simulink library "GearLibrary"  (R2017b)
settings: Solver=VariableStepAuto  StartTime=0.0  StopTime=10.0  RelTol=1e-3
undefined symbols (not defined in the file): c_LTset, DiscIntNeverNeededParam, g, Gear, magnitude, Strut, Tss, x1_LTset
libraries: GearLibrary x11, BaseLibrary x6, simulink x4, MathLibrary x2, vrlib x1
(part 1 of 2)
settings Model: Creator=Holzapfel  LastModifiedBy=zht
settings CodeAppCC: StateflowObjectComments=on

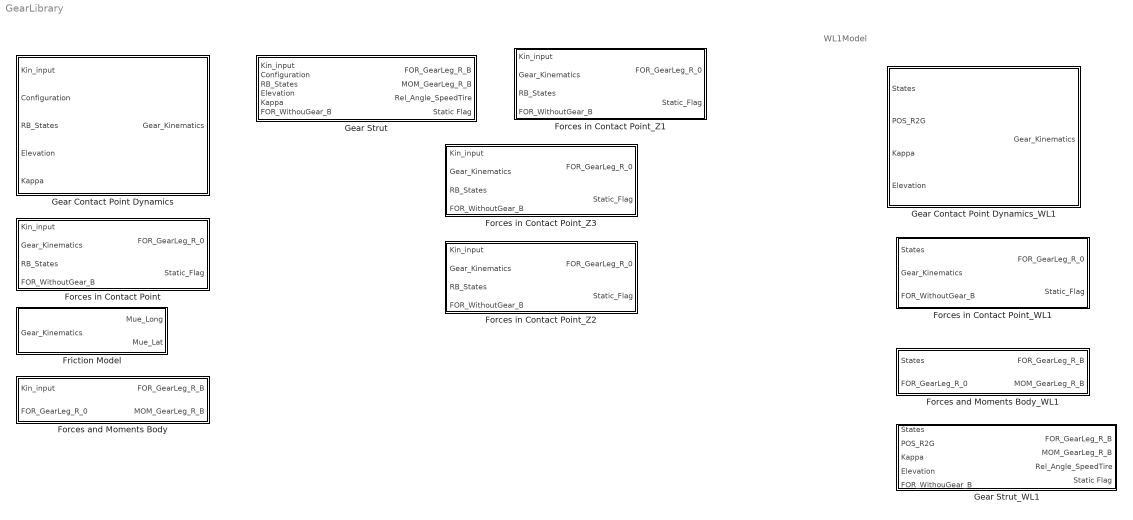
== system GearLibrary ==
  note: WL1Model
  Forces and Moments Body : Subsystem  mask{POS_R_GearStrut_B=Strut.POS_R_GearStrut_B}
      mask prompts: POS_R_GearStrut_B "POS R => Contact Point, Body Frame"
  Forces and Moments Body_WL1 : Subsystem  mask{POS_R_GearStrut_B=Strut.POS_R_GearStrut_B}
      mask prompts: POS_R_GearStrut_B "POS R => Contact Point, Body Frame"
  Forces in Contact Point : Subsystem  mask{h_StrutUndeflected=Strut.h_StrutUndeflected, c=Strut.c, d=Strut.d, ct=Strut.ct, dt=Strut.dt, FOR_MaxDamp=Strut.FOR_MaxDamp, FOR_MaxSpring=Strut.FOR_MaxSpring, Mue_Roll=Strut.Mue_Roll, Mue_Lat_per_Slip=Strut.Mue_Lat_per_Slip, Mue_Lat_Max=Strut.Mue_Lat_Max, Compress_LengthMax=Strut.Compress_LengthMax, Mue_Static=Strut.Mue_Static}
      mask prompts: h_StrutUndeflected "Length of undeflected landing gear strut [m]"; c "Strut Spring Constant [N/m]"; d "Strut Damping Constant [N/(m/s)]"; ct "Consider tire and ground is also a spring system, so it's Ground Spring Constant [N/m]"; dt "Consider tire and ground is also a spring system, so it's Ground Damping Constant [N/m]"; FOR_MaxDamp "Maximum Strut Damper Force [N]"; FOR_MaxSpring "Maximum Strut Spring Force [Nm]"; Mue_Roll "Rolling Friction Coefficient [-]"; Mue_Lat_per_Slip "Lateral Friction Coefficient per Slip Angle [1/rad]"; Mue_Lat_Max "Maximum Lateral Friction Coefficient [-]"; Compress_LengthMax "Maximum Compression length [m]"; Mue_Static "Static  Friction Coefficient"
  Forces in Contact Point_WL1 : Subsystem  mask{h_StrutUndeflected=Strut.h_StrutUndeflected, c=Strut.c, d=Strut.d, ct=Strut.ct, dt=Strut.dt, FOR_MaxDamp=Strut.FOR_MaxDamp, FOR_MaxSpring=Strut.FOR_MaxSpring, Mue_Roll=Strut.Mue_Roll, Mue_Lat_per_Slip=Strut.Mue_Lat_per_Slip, Mue_Lat_Max=Strut.Mue_Lat_Max, Compress_LengthMax=Strut.Compress_LengthMax, Mue_Static=Strut.Mue_Static, Compress_LengthMax_Tire=Strut.Compress_LengthMax_Tire}
      mask prompts: h_StrutUndeflected "Length of undeflected landing gear strut [m]"; c "Strut Spring Constant [N/m]"; d "Strut Damping Constant [N/(m/s)]"; ct "Consider tire and ground is also a spring system, so it's Ground Spring Constant [N/m]"; dt "Consider tire and ground is also a spring system, so it's Ground Damping Constant [N/m]"; FOR_MaxDamp "Maximum Strut Damper Force [N]"; FOR_MaxSpring "Maximum Strut Spring Force [Nm]"; Mue_Roll "Rolling Friction Coefficient [-]"; Mue_Lat_per_Slip "Lateral Friction Coefficient per Slip Angle [1/rad]"; Mue_Lat_Max "Maximum Lateral Friction Coefficient [-]"; Compress_LengthMax "Maximum Compression length [m]"; Mue_Static "Static  Friction Coefficient"; Compress_LengthMax_Tire "Maximum Compression length [m]"
  Forces in Contact Point_Z1 : Subsystem  mask{h_StrutUndeflected=Strut.h_StrutUndeflected, c=Strut.c, d=Strut.d, ct=Strut.ct, dt=Strut.dt, FOR_MaxDamp=Strut.FOR_MaxDamp, FOR_MaxSpring=Strut.FOR_MaxSpring, Mue_Roll=Strut.Mue_Roll, Mue_Lat_per_Slip=Strut.Mue_Lat_per_Slip, Mue_Lat_Max=Strut.Mue_Lat_Max, Compress_LengthMax=Strut.Compress_LengthMax, Mue_Static=Strut.Mue_Static, Compress_LengthMax_Tire=Strut.Compress_LengthMax_Tire}
      mask prompts: h_StrutUndeflected "Length of undeflected landing gear strut [m]"; c "Strut Spring Constant [N/m]"; d "Strut Damping Constant [N/(m/s)]"; ct "Consider tire and ground is also a spring system, so it's Ground Spring Constant [N/m]"; dt "Consider tire and ground is also a spring system, so it's Ground Damping Constant [N/m]"; FOR_MaxDamp "Maximum Strut Damper Force [N]"; FOR_MaxSpring "Maximum Strut Spring Force [Nm]"; Mue_Roll "Rolling Friction Coefficient [-]"; Mue_Lat_per_Slip "Lateral Friction Coefficient per Slip Angle [1/rad]"; Mue_Lat_Max "Maximum Lateral Friction Coefficient [-]"; Compress_LengthMax "Maximum Compression length [m]"; Mue_Static "Static  Friction Coefficient"; Compress_LengthMax_Tire "Maximum Compression length [m]"
  Forces in Contact Point_Z2 : Subsystem  mask{h_StrutUndeflected=Strut.h_StrutUndeflected, c=Strut.c, d=Strut.d, ct=Strut.ct, dt=Strut.dt, FOR_MaxDamp=Strut.FOR_MaxDamp, FOR_MaxSpring=Strut.FOR_MaxSpring, Mue_Roll=Strut.Mue_Roll, Mue_Lat_per_Slip=Strut.Mue_Lat_per_Slip, Mue_Lat_Max=Strut.Mue_Lat_Max, Compress_LengthMax=Strut.Compress_LengthMax, Mue_Static=Strut.Mue_Static, Compress_LengthMax_Tire=Strut.Compress_LengthMax_Tire}
      mask prompts: h_StrutUndeflected "Length of undeflected landing gear strut [m]"; c "Strut Spring Constant [N/m]"; d "Strut Damping Constant [N/(m/s)]"; ct "Consider tire and ground is also a spring system, so it's Ground Spring Constant [N/m]"; dt "Consider tire and ground is also a spring system, so it's Ground Damping Constant [N/m]"; FOR_MaxDamp "Maximum Strut Damper Force [N]"; FOR_MaxSpring "Maximum Strut Spring Force [Nm]"; Mue_Roll "Rolling Friction Coefficient [-]"; Mue_Lat_per_Slip "Lateral Friction Coefficient per Slip Angle [1/rad]"; Mue_Lat_Max "Maximum Lateral Friction Coefficient [-]"; Compress_LengthMax "Maximum Compression length [m]"; Mue_Static "Static  Friction Coefficient"; Compress_LengthMax_Tire "Maximum Compression length [m]"
  Forces in Contact Point_Z3 : Subsystem  mask{h_StrutUndeflected=Strut.h_StrutUndeflected, c=Strut.c, d=Strut.d, ct=Strut.ct, dt=Strut.dt, FOR_MaxDamp=Strut.FOR_MaxDamp, FOR_MaxSpring=Strut.FOR_MaxSpring, Mue_Roll=Strut.Mue_Roll, Mue_Lat_per_Slip=Strut.Mue_Lat_per_Slip, Mue_Lat_Max=Strut.Mue_Lat_Max, Compress_LengthMax=Strut.Compress_LengthMax, Mue_Static=Strut.Mue_Static}
      mask prompts: h_StrutUndeflected "Length of undeflected landing gear strut [m]"; c "Strut Spring Constant [N/m]"; d "Strut Damping Constant [N/(m/s)]"; ct "Consider tire and ground is also a spring system, so it's Ground Spring Constant [N/m]"; dt "Consider tire and ground is also a spring system, so it's Ground Damping Constant [N/m]"; FOR_MaxDamp "Maximum Strut Damper Force [N]"; FOR_MaxSpring "Maximum Strut Spring Force [Nm]"; Mue_Roll "Rolling Friction Coefficient [-]"; Mue_Lat_per_Slip "Lateral Friction Coefficient per Slip Angle [1/rad]"; Mue_Lat_Max "Maximum Lateral Friction Coefficient [-]"; Compress_LengthMax "Maximum Compression length [m]"; Mue_Static "Static  Friction Coefficient"
  Friction Model : Subsystem  mask{Mue_Roll=Strut.Mue_Roll, Mue_Lat_per_Slip=Strut.Mue_Lat_per_Slip, Mue_Lat_Max=Strut.Mue_Lat_Max}
      mask prompts: Mue_Roll "Rolling friction coefficient [-]"; Mue_Lat_per_Slip "Lateral friction coefficient per Slip Angle [1/rad]"; Mue_Lat_Max "Maximum Lateral Friction Coefficient [-]"
  Gear Contact Point Dynamics : Subsystem  mask{POS_R_GearStrut_B=Strut.POS_R_GearStrut_B}
      mask prompts: POS_R_GearStrut_B "POS R => Gear Contact Pt., Body Frame"
  Gear Contact Point Dynamics_WL1 : Subsystem  mask{POS_R_GearStrut_B=Strut.POS_R_GearStrut_B}
      mask prompts: POS_R_GearStrut_B "POS R => Gear Contact Pt., Body Frame"
  Gear Strut : Subsystem  mask{Strut=Gear.NoseStrut}
      mask prompts: Strut "Landing Gear Strut Structure"
  Gear Strut_WL1 : Subsystem  mask{Strut=Gear.NoseStrut}
      mask prompts: Strut "Landing Gear Strut Structure"

== system GearLibrary/Forces and Moments Body ==
  Kin_input : Inport  OutDataTypeStr=Bus: Kin_input_BUS
  "FOR_GearLeg_R_0 " : Inport  Port=2  Unit=N  PortDimensions=[3,1]
  Bus Selector : BusSelector  OutputSignals=M_BO
  Compute Gear Moment : BaseLibrary/CrossProduct
  Lever Arm R=>GearContact Point : Constant  Value=POS_R_GearStrut_B  VectorParams1D=off
  Product : Product  Multiplication=Matrix(*)
  FOR_GearLeg_R_B : Outport  Unit=N  PortDimensions=[3,1]
  MOM_GearLeg_R_B : Outport  Port=2  Unit=N*m  PortDimensions=[3,1]
  wires:
  Kin_input/1 -> Bus Selector/1
  Compute Gear Moment/1 -> MOM_GearLeg_R_B/1
  Lever Arm R=>GearContact Point/1 -> Compute Gear Moment/1
  Bus Selector/1 -> Product/1  "<M_BO>"
  "FOR_GearLeg_R_0 "/1 -> Product/2
  Product/1 -> Compute Gear Moment/2, FOR_GearLeg_R_B/1

== system GearLibrary/Forces and Moments Body_WL1 ==
  States : Inport  OutDataTypeStr=Bus: States_BUS
  "FOR_GearLeg_R_0 " : Inport  Port=2  Unit=N  PortDimensions=[3,1]
  Bus Selector : BusSelector  OutputSignals=M_BE
  Compute Gear Moment : MathLibrary/CrossProduct
  Lever Arm R=>GearContact Point : Constant  Value=POS_R_GearStrut_B  VectorParams1D=off
  Product : Product  Multiplication=Matrix(*)
  FOR_GearLeg_R_B : Outport  Unit=N  PortDimensions=[3,1]
  MOM_GearLeg_R_B : Outport  Port=2  Unit=N*m  PortDimensions=[3,1]
  wires:
  States/1 -> Bus Selector/1
  Compute Gear Moment/1 -> MOM_GearLeg_R_B/1
  Lever Arm R=>GearContact Point/1 -> Compute Gear Moment/1
  Bus Selector/1 -> Product/1  "<M_BE>"
  "FOR_GearLeg_R_0 "/1 -> Product/2
  Product/1 -> Compute Gear Moment/2, FOR_GearLeg_R_B/1

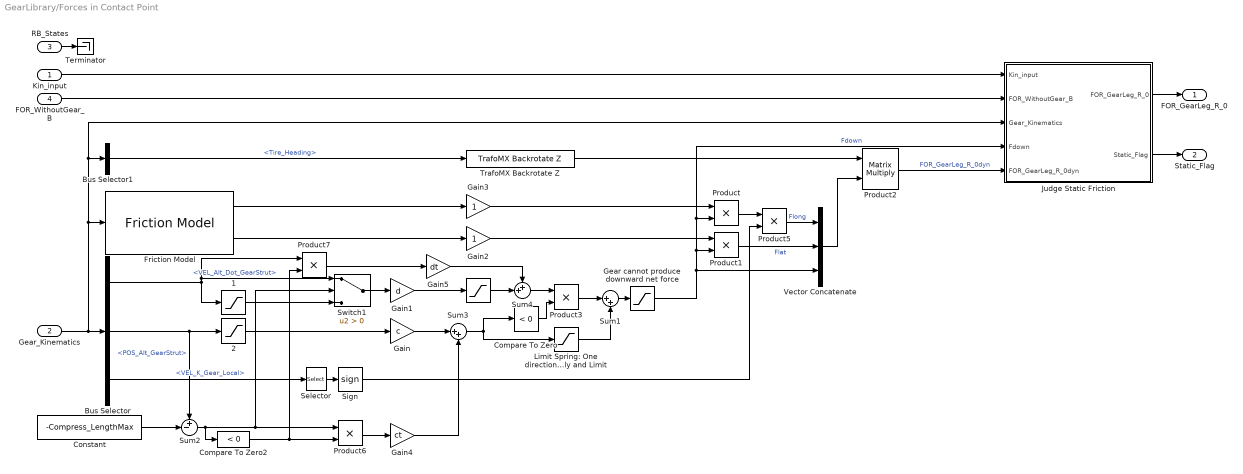
== system GearLibrary/Forces in Contact Point ==
  Kin_input : Inport  OutDataTypeStr=Bus: Kin_input_BUS
  Gear_Kinematics : Inport  Port=2  OutDataTypeStr=Bus: GearKinematics_BUS
  RB_States : Inport  Port=3  OutDataTypeStr=Bus: RB_State_BUS
  FOR_WithoutGear_B : Inport  Port=4  Unit=N  PortDimensions=[3 1]
  " " : Saturate  UpperLimit=FOR_MaxDamp  LowerLimit=-FOR_MaxDamp
  " 1" : Saturate  UpperLimit=inf  LowerLimit=0
  " 2" : Saturate  UpperLimit=0  LowerLimit=-Compress_LengthMax
  " Sign " : Signum
  Bus Selector : BusSelector  OutputSignals=VEL_Alt_Dot_GearStrut,POS_Alt_GearStrut,VEL_K_Gear_Local
  Bus Selector1 : BusSelector  OutputSignals=Tire_Heading
  Compare To Zero : simulink/Logic and Bit Operations/Compare To Zero  relop=<  OutDataTypeStr=boolean
  Compare To Zero2 : simulink/Logic and Bit Operations/Compare To Zero  relop=<  OutDataTypeStr=boolean
  Constant : Constant  Value=-Compress_LengthMax
  Friction Model : GearLibrary/Friction Model  Mue_Roll=Strut.Mue_Roll  Mue_Lat_per_Slip=Strut.Mue_Lat_per_Slip  Mue_Lat_Max=Strut.Mue_Lat_Max
  Gain : Gain  Gain=c
  Gain1 : Gain  Gain=d
  Gain2 : Gain
  Gain3 : Gain
  Gain4 : Gain  Gain=ct
  Gain5 : Gain  Gain=dt
  Gear cannot produce downward net force : Saturate  UpperLimit=0  LowerLimit=-inf
  Judge Static Friction : Subsystem
  Limit Spring: One direction only and Limit : Saturate  UpperLimit=0  LowerLimit=-FOR_MaxSpring
  Product{,1,3,5..7} (6 alike) : Product
  Product2 : Product  Multiplication=Matrix(*)
  Selector : Selector  InputPortWidth=3  IndexOptions=Index vector (dialog)  Indices=[1]  OutputSizes=1
  Sum1 : Sum  Inputs=|++
  Sum2 : Sum  Inputs=+-|
  Sum3 : Sum  Inputs=|++
  Sum4 : Sum  Inputs=++|
  Switch1 : Switch  Criteria=u2 > Threshold
  Terminator : Terminator
  TrafoMX Backrotate Z : BaseLibrary/TrafoMX Backrotate Z
  Vector Concatenate : Concatenate  NumInputs=3  Mode=Multidimensional array
  FOR_GearLeg_R_0 : Outport  Unit=N  PortDimensions=[3,1]
  Static_Flag : Outport  Port=2  PortDimensions=[1]
  wires:
  Friction Model/1 -> Gain3/1
  Friction Model/2 -> Gain2/1
  Compare To Zero/1 -> Product3/2
  Limit Spring: One direction only and Limit/1 -> Sum1/2
  Product3/1 -> Sum1/1
  Vector Concatenate/1 -> Product2/2
  TrafoMX Backrotate Z/1 -> Product2/1
  Bus Selector1/1 -> TrafoMX Backrotate Z/1  "<Tire_Heading>"
  Sum1/1 -> Gear cannot produce downward net force/1
  Gain1/1 -> " "/1
  Bus Selector/2 -> " 2"/1, Sum2/1  "<POS_Alt_GearStrut>"
  Gain3/1 -> Product/1
  Gain2/1 -> Product1/1
  Sum2/1 -> Compare To Zero2/1, Product6/1, Switch1/2
  Constant/1 -> Sum2/2
  " 2"/1 -> Gain/1
  Bus Selector/1 -> Product7/1, Switch1/1, " 1"/1  "<VEL_Alt_Dot_GearStrut>"
  Switch1/1 -> Gain1/1
  " 1"/1 -> Switch1/3
  Compare To Zero2/1 -> Product6/2, Product7/2
  Product6/1 -> Gain4/1
  Gain4/1 -> Sum3/2
  Gain/1 -> Sum3/1
  Sum3/1 -> Limit Spring: One direction only and Limit/1, Compare To Zero/1
  Product7/1 -> Gain5/1
  Gain5/1 -> Sum4/1
  " "/1 -> Sum4/2
  Sum4/1 -> Product3/1
  Bus Selector/3 -> Selector/1  "<VEL_K_Gear_Local>"
  Product2/1 -> Judge Static Friction/5(FOR_GearLeg_R_0dyn)  "FOR_GearLeg_R_0dyn"
  Selector/1 -> " Sign "/1
  Product1/1 -> Vector Concatenate/2  "Flat"
  Gear cannot produce downward net force/1 -> Product/2, Judge Static Friction/4(Fdown), Product1/2, Vector Concatenate/3  "Fdown"
  Product/1 -> Product5/1
  Product5/1 -> Vector Concatenate/1  "Flong"
  " Sign "/1 -> Product5/2
  RB_States/1 -> Terminator/1
  FOR_WithoutGear_B/1 -> Judge Static Friction/2(FOR_WithoutGear_B)
  Kin_input/1 -> Judge Static Friction/1(Kin_input)
  Gear_Kinematics/1 -> Judge Static Friction/3(Gear_Kinematics), Bus Selector1/1, Friction Model/1, Bus Selector/1
  Judge Static Friction/1(FOR_GearLeg_R_0) -> FOR_GearLeg_R_0/1
  Judge Static Friction/2(Static_Flag) -> Static_Flag/1

== system GearLibrary/Forces in Contact Point_WL1 ==
  States : Inport  OutDataTypeStr=Bus: States_BUS
  Gear_Kinematics : Inport  Port=2  OutDataTypeStr=Bus: GearKinematics_BUS
  FOR_WithoutGear_B : Inport  Port=3  Unit=N  PortDimensions=[3 1]
  " Sign " : Signum
  Bus Selector : BusSelector  OutputSignals=VEL_K_Gear_Local,VEL_Alt_Dot_GearStrut,POS_Alt_GearStrut
  Bus Selector1 : BusSelector  OutputSignals=Tire_Heading
  Constant : Constant  Value=Compress_LengthMax
  Friction Model : GearLibrary/Friction Model  Mue_Roll=Strut.Mue_Roll  Mue_Lat_per_Slip=Strut.Mue_Lat_per_Slip  Mue_Lat_Max=Strut.Mue_Lat_Max
  Gain1 : Gain
  Gain3 : Gain
  If : If  NumInputs=2  IfExpression=u1 >= 0  ElseIfExpressions=u1 < 0 & u1 >= (-u2)
  If Action Subsystem : Subsystem  TreatAsAtomicUnit=on
  If Action Subsystem1 : Subsystem  TreatAsAtomicUnit=on
  If Action Subsystem2 : Subsystem  TreatAsAtomicUnit=on
  Judge Static Friction : Subsystem
  Merge : Merge  Inputs=3
  Product : Product
  Product1 : Product
  Product2 : Product  Multiplication=Matrix(*)
  Product5 : Product
  Selector : Selector  InputPortWidth=3  IndexOptions=Index vector (dialog)  Indices=[1]  OutputSizes=1
  TrafoMX Backrotate Z : MathLibrary/Backrotate Z
  Vector Concatenate : Concatenate  NumInputs=3  Mode=Multidimensional array
  FOR_GearLeg_R_0 : Outport  Unit=N  PortDimensions=[3,1]
  Static_Flag : Outport  Port=2  PortDimensions=[1]
  wires:
  Constant/1 -> If/2
  Bus Selector/3 -> If Action Subsystem1/2(x), If Action Subsystem2/2(x), If/1  "<POS_Alt_GearStrut>"
  Bus Selector/2 -> If Action Subsystem1/1(v), If Action Subsystem2/1(v)  "<VEL_Alt_Dot_GearStrut>"
  If Action Subsystem/1(Fz=0) -> Merge/1
  If/1 -> If Action Subsystem/Action
  If Action Subsystem2/1(Fz) -> Merge/3  "Fz2"
  If Action Subsystem1/1(Fz) -> Merge/2  "Fz1"
  If/2 -> If Action Subsystem1/Action
  If/3 -> If Action Subsystem2/Action
  Friction Model/1 -> Gain3/1
  Friction Model/2 -> Gain1/1
  Vector Concatenate/1 -> Product2/2
  TrafoMX Backrotate Z/1 -> Product2/1
  Bus Selector1/1 -> TrafoMX Backrotate Z/1  "<Tire_Heading>"
  Gain3/1 -> Product/1
  Gain1/1 -> Product1/1
  Bus Selector/1 -> Selector/1  "<VEL_K_Gear_Local>"
  Product2/1 -> Judge Static Friction/5(FOR_GearLeg_R_0dyn)  "FOR_GearLeg_R_0dyn"
  Selector/1 -> " Sign "/1
  Product1/1 -> Vector Concatenate/2  "Flat"
  Merge/1 -> Product/2, Judge Static Friction/4(Fdown), Product1/2, Vector Concatenate/3  "Fdown"
  Product/1 -> Product5/1
  Product5/1 -> Vector Concatenate/1  "Flong"
  " Sign "/1 -> Product5/2
  FOR_WithoutGear_B/1 -> Judge Static Friction/2(FOR_WithoutGear_B)
  States/1 -> Judge Static Friction/1(States)
  Gear_Kinematics/1 -> Judge Static Friction/3(Gear_Kinematics), Bus Selector1/1, Friction Model/1, Bus Selector/1
  Judge Static Friction/1(FOR_GearLeg_R_0) -> FOR_GearLeg_R_0/1
  Judge Static Friction/2(Static_Flag) -> Static_Flag/1

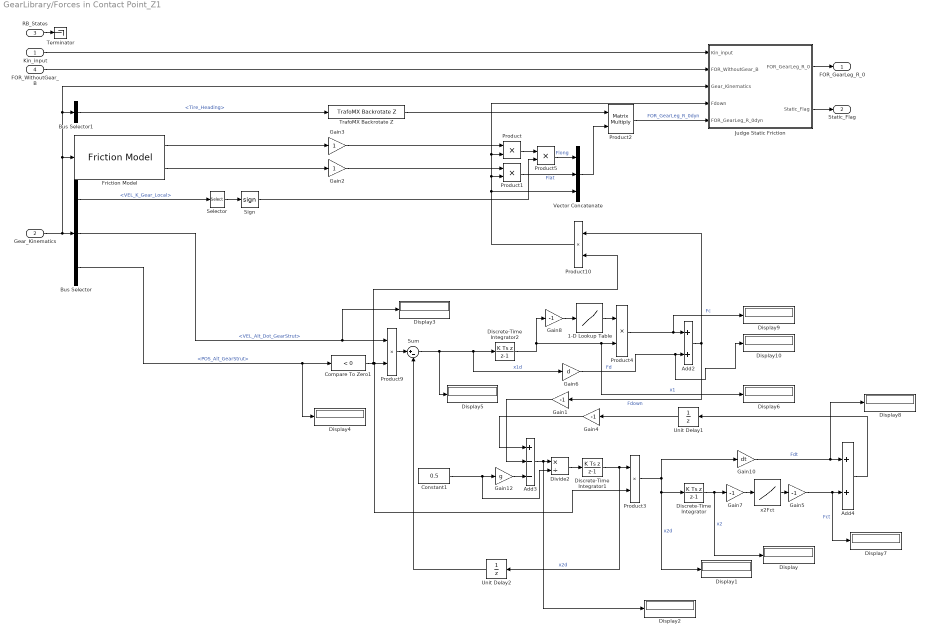
== system GearLibrary/Forces in Contact Point_Z1 ==
  Kin_input : Inport  OutDataTypeStr=Bus: Kin_input_BUS
  Gear_Kinematics : Inport  Port=2  OutDataTypeStr=Bus: GearKinematics_BUS
  RB_States : Inport  Port=3  OutDataTypeStr=Bus: RB_State_BUS
  FOR_WithoutGear_B : Inport  Port=4  Unit=N  PortDimensions=[3 1]
  " Sign " : Signum
  1-D Lookup Table : Lookup_n-D  NumberOfTableDimensions=1  BreakpointsForDimension1=[0,linspace(Compress_LengthMax,Compress_LengthMax+0.001,29)]  Table=[c,linspace(c,c*20,29)]  InternalRulePriority=Speed  RndMeth=Simplest  InputSameDT=on
  Add2 : Sum
  Add3 : Sum  Inputs=+--
  Add4 : Sum
  Bus Selector : BusSelector  OutputSignals=VEL_K_Gear_Local,VEL_Alt_Dot_GearStrut,POS_Alt_GearStrut
  Bus Selector1 : BusSelector  OutputSignals=Tire_Heading
  Compare To Zero1 : simulink/Logic and Bit Operations/Compare To Zero  relop=<  OutDataTypeStr=boolean
  Constant1 : Constant  Value=0.5  SampleTime=Tss
  Discrete-Time Integrator : DiscreteIntegrator  IntegratorMethod=Integration: Backward Euler  InitialConditionSetting=State (most efficient)  SampleTime=Tss  LimitOutput=on  UpperSaturationLimit=0  ICPrevOutput=DiscIntNeverNeededParam  ICPrevScaledInput=DiscIntNeverNeededParam
  Discrete-Time Integrator1 : DiscreteIntegrator  IntegratorMethod=Integration: Backward Euler  InitialConditionSetting=State (most efficient)  SampleTime=Tss  ICPrevOutput=DiscIntNeverNeededParam  ICPrevScaledInput=DiscIntNeverNeededParam
  Discrete-Time Integrator2 : DiscreteIntegrator  IntegratorMethod=Integration: Backward Euler  InitialConditionSetting=State (most efficient)  SampleTime=Tss  ICPrevOutput=DiscIntNeverNeededParam  ICPrevScaledInput=DiscIntNeverNeededParam
  Display{,1..10} (11 alike) : Display
  Divide2 : Product  Inputs=*/
  Friction Model : GearLibrary/Friction Model  Mue_Roll=Strut.Mue_Roll  Mue_Lat_per_Slip=Strut.Mue_Lat_per_Slip  Mue_Lat_Max=Strut.Mue_Lat_Max
  Gain{1,4..5,7..8} (5 alike) : Gain  Gain=-1
  Gain10 : Gain  Gain=dt
  Gain12 : Gain  Gain=g
  Gain2 : Gain
  Gain3 : Gain
  Gain6 : Gain  Gain=d
  Judge Static Friction : Subsystem
  Product{,1,3..5,9..10} (7 alike) : Product
  Product2 : Product  Multiplication=Matrix(*)
  Selector : Selector  InputPortWidth=3  IndexOptions=Index vector (dialog)  Indices=[1]  OutputSizes=1
  Sum : Sum  Inputs=|+-
  Terminator : Terminator
  TrafoMX Backrotate Z : BaseLibrary/TrafoMX Backrotate Z
  Unit Delay1 : UnitDelay  SampleTime=-1
  Unit Delay2 : UnitDelay  SampleTime=-1
  Vector Concatenate : Concatenate  NumInputs=3  Mode=Multidimensional array
  x2Fct : Lookup_n-D  NumberOfTableDimensions=1  BreakpointsForDimension1=linspace(0,Compress_LengthMax_Tire,30)  Table=(linspace(0,Compress_LengthMax_Tire,30) * (9 * ct / Compress_LengthMax_Tire) + ct).*linspace(0,Compress_LengthMax_Tire,30)  InternalRulePriority=Speed  RndMeth=Simplest  InputSameDT=on
  FOR_GearLeg_R_0 : Outport  Unit=N  PortDimensions=[3,1]
  Static_Flag : Outport  Port=2  PortDimensions=[1]
  wires:
  Friction Model/1 -> Gain3/1
  Friction Model/2 -> Gain2/1
  Vector Concatenate/1 -> Product2/2
  TrafoMX Backrotate Z/1 -> Product2/1
  Bus Selector1/1 -> TrafoMX Backrotate Z/1  "<Tire_Heading>"
  Gain3/1 -> Product/1
  Gain2/1 -> Product1/1
  Bus Selector/1 -> Selector/1  "<VEL_K_Gear_Local>"
  Product2/1 -> Judge Static Friction/5(FOR_GearLeg_R_0dyn)  "FOR_GearLeg_R_0dyn"
  Selector/1 -> " Sign "/1
  Product1/1 -> Vector Concatenate/2  "Flat"
  Add2/1 -> Product10/1, Gain1/1  "Fdown"
  Product/1 -> Product5/1
  Product5/1 -> Vector Concatenate/1  "Flong"
  " Sign "/1 -> Product5/2
  RB_States/1 -> Terminator/1
  FOR_WithoutGear_B/1 -> Judge Static Friction/2(FOR_WithoutGear_B)
  Kin_input/1 -> Judge Static Friction/1(Kin_input)
  Gear_Kinematics/1 -> Judge Static Friction/3(Gear_Kinematics), Bus Selector1/1, Friction Model/1, Bus Selector/1
  Judge Static Friction/1(FOR_GearLeg_R_0) -> FOR_GearLeg_R_0/1
  Judge Static Friction/2(Static_Flag) -> Static_Flag/1
  Constant1/1 -> Divide2/2, Gain12/1
  Sum/1 -> Display5/1, Discrete-Time Integrator2/1, Gain6/1  "x1d"
  Bus Selector/2 -> Display3/1, Product9/1  "<VEL_Alt_Dot_GearStrut>"
  Bus Selector/3 -> Display4/1, Compare To Zero1/1  "<POS_Alt_GearStrut>"
  Product4/1 -> Display9/1, Add2/1  "Fc"
  Gain8/1 -> 1-D Lookup Table/1
  Product3/1 -> Gain10/1, Display1/1, Discrete-Time Integrator/1  "x2d"
  Product9/1 -> Sum/1
  x2Fct/1 -> Gain5/1
  Add3/1 -> Display2/1, Divide2/1
  Discrete-Time Integrator2/1 -> Display6/1, Product4/2, Gain8/1  "x1"
  Discrete-Time Integrator/1 -> Gain7/1, Display/1  "x2"
  Compare To Zero1/1 -> Product10/2, Product3/2, Product9/2
  Gain10/1 -> Display8/1, Add4/1  "Fdt"
  Gain12/1 -> Add3/3
  1-D Lookup Table/1 -> Product4/1
  Gain6/1 -> Display10/1, Add2/2  "Fd"
  Product10/1 -> Product/2, Judge Static Friction/4(Fdown), Product1/2, Vector Concatenate/3
  Add4/1 -> Unit Delay1/1
  Unit Delay1/1 -> Gain4/1
  Unit Delay2/1 -> Sum/2
  Divide2/1 -> Discrete-Time Integrator1/1
  Discrete-Time Integrator1/1 -> Unit Delay2/1, Product3/1  "x2d"
  Gain1/1 -> Add3/2
  Gain4/1 -> Add3/1
  Gain5/1 -> Display7/1, Add4/2  "Fct"
  Gain7/1 -> x2Fct/1

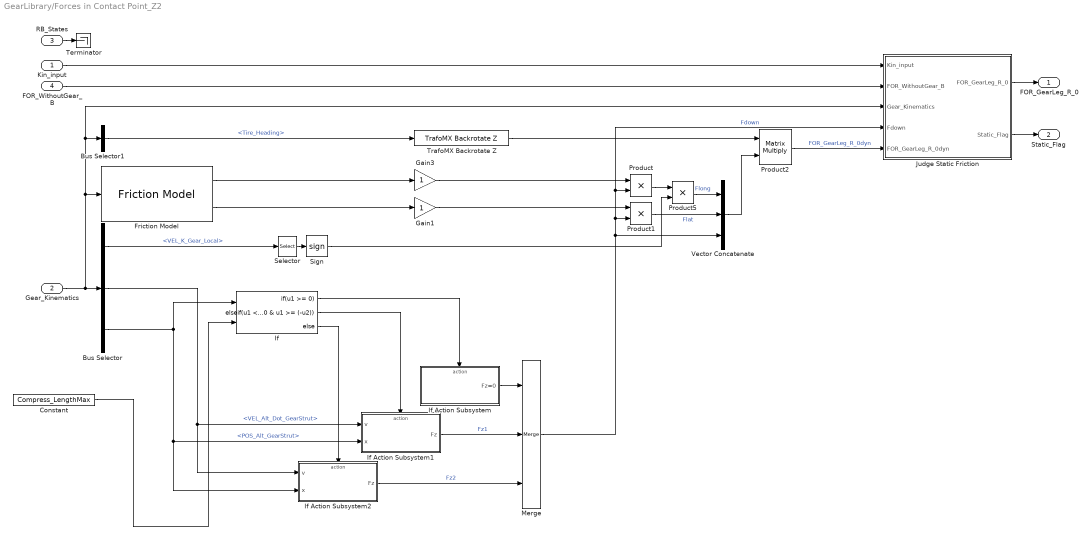
== system GearLibrary/Forces in Contact Point_Z2 ==
  Kin_input : Inport  OutDataTypeStr=Bus: Kin_input_BUS
  Gear_Kinematics : Inport  Port=2  OutDataTypeStr=Bus: GearKinematics_BUS
  RB_States : Inport  Port=3  OutDataTypeStr=Bus: RB_State_BUS
  FOR_WithoutGear_B : Inport  Port=4  Unit=N  PortDimensions=[3 1]
  " Sign " : Signum
  Bus Selector : BusSelector  OutputSignals=VEL_K_Gear_Local,VEL_Alt_Dot_GearStrut,POS_Alt_GearStrut
  Bus Selector1 : BusSelector  OutputSignals=Tire_Heading
  Constant : Constant  Value=Compress_LengthMax
  Friction Model : GearLibrary/Friction Model  Mue_Roll=Strut.Mue_Roll  Mue_Lat_per_Slip=Strut.Mue_Lat_per_Slip  Mue_Lat_Max=Strut.Mue_Lat_Max
  Gain1 : Gain
  Gain3 : Gain
  If : If  NumInputs=2  IfExpression=u1 >= 0  ElseIfExpressions=u1 < 0 & u1 >= (-u2)
  If Action Subsystem : Subsystem  TreatAsAtomicUnit=on
  If Action Subsystem1 : Subsystem  TreatAsAtomicUnit=on
  If Action Subsystem2 : Subsystem  TreatAsAtomicUnit=on
  Judge Static Friction : Subsystem
  Merge : Merge  Inputs=3
  Product : Product
  Product1 : Product
  Product2 : Product  Multiplication=Matrix(*)
  Product5 : Product
  Selector : Selector  InputPortWidth=3  IndexOptions=Index vector (dialog)  Indices=[1]  OutputSizes=1
  Terminator : Terminator
  TrafoMX Backrotate Z : BaseLibrary/TrafoMX Backrotate Z
  Vector Concatenate : Concatenate  NumInputs=3  Mode=Multidimensional array
  FOR_GearLeg_R_0 : Outport  Unit=N  PortDimensions=[3,1]
  Static_Flag : Outport  Port=2  PortDimensions=[1]
  wires:
  Judge Static Friction/2(Static_Flag) -> Static_Flag/1
  Judge Static Friction/1(FOR_GearLeg_R_0) -> FOR_GearLeg_R_0/1
  Gear_Kinematics/1 -> Bus Selector/1, Friction Model/1, Bus Selector1/1, Judge Static Friction/3(Gear_Kinematics)
  Kin_input/1 -> Judge Static Friction/1(Kin_input)
  FOR_WithoutGear_B/1 -> Judge Static Friction/2(FOR_WithoutGear_B)
  RB_States/1 -> Terminator/1
  " Sign "/1 -> Product5/2
  Product5/1 -> Vector Concatenate/1  "Flong"
  Product/1 -> Product5/1
  Merge/1 -> Vector Concatenate/3, Product1/2, Judge Static Friction/4(Fdown), Product/2  "Fdown"
  Product1/1 -> Vector Concatenate/2  "Flat"
  Selector/1 -> " Sign "/1
  Product2/1 -> Judge Static Friction/5(FOR_GearLeg_R_0dyn)  "FOR_GearLeg_R_0dyn"
  Bus Selector/1 -> Selector/1  "<VEL_K_Gear_Local>"
  Gain1/1 -> Product1/1
  Gain3/1 -> Product/1
  Bus Selector1/1 -> TrafoMX Backrotate Z/1  "<Tire_Heading>"
  TrafoMX Backrotate Z/1 -> Product2/1
  Vector Concatenate/1 -> Product2/2
  Friction Model/2 -> Gain1/1
  Friction Model/1 -> Gain3/1
  If/3 -> If Action Subsystem2/Action
  If/2 -> If Action Subsystem1/Action
  If Action Subsystem1/1(Fz) -> Merge/2  "Fz1"
  If Action Subsystem2/1(Fz) -> Merge/3  "Fz2"
  If/1 -> If Action Subsystem/Action
  If Action Subsystem/1(Fz=0) -> Merge/1
  Bus Selector/2 -> If Action Subsystem2/1(v), If Action Subsystem1/1(v)  "<VEL_Alt_Dot_GearStrut>"
  Bus Selector/3 -> If/1, If Action Subsystem2/2(x), If Action Subsystem1/2(x)  "<POS_Alt_GearStrut>"
  Constant/1 -> If/2

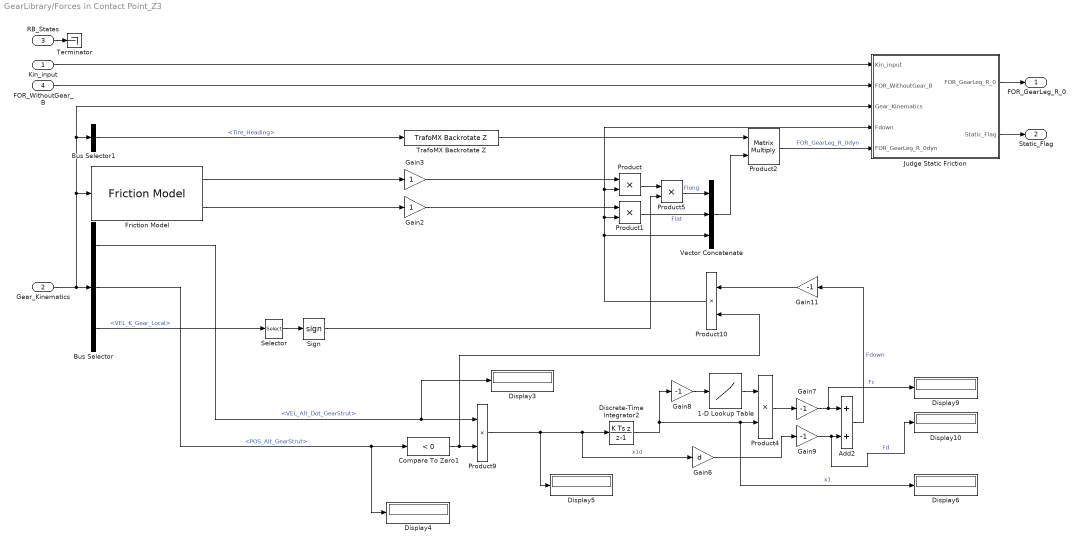
== system GearLibrary/Forces in Contact Point_Z3 ==
  Kin_input : Inport  OutDataTypeStr=Bus: Kin_input_BUS
  Gear_Kinematics : Inport  Port=2  OutDataTypeStr=Bus: GearKinematics_BUS
  RB_States : Inport  Port=3  OutDataTypeStr=Bus: RB_State_BUS
  FOR_WithoutGear_B : Inport  Port=4  Unit=N  PortDimensions=[3 1]
  " Sign " : Signum
  1-D Lookup Table : Lookup_n-D  NumberOfTableDimensions=1  BreakpointsForDimension1=x1_LTset  Table=c_LTset  InternalRulePriority=Speed  RndMeth=Simplest  InputSameDT=on
  Add2 : Sum
  Bus Selector : BusSelector  OutputSignals=VEL_Alt_Dot_GearStrut,POS_Alt_GearStrut,VEL_K_Gear_Local
  Bus Selector1 : BusSelector  OutputSignals=Tire_Heading
  Compare To Zero1 : simulink/Logic and Bit Operations/Compare To Zero  relop=<  OutDataTypeStr=boolean
  Discrete-Time Integrator2 : DiscreteIntegrator  IntegratorMethod=Integration: Backward Euler  InitialConditionSetting=State (most efficient)  SampleTime=Tss  ICPrevOutput=DiscIntNeverNeededParam  ICPrevScaledInput=DiscIntNeverNeededParam
  Display{3..6,9..10} (6 alike) : Display
  Friction Model : GearLibrary/Friction Model  Mue_Roll=Strut.Mue_Roll  Mue_Lat_per_Slip=Strut.Mue_Lat_per_Slip  Mue_Lat_Max=Strut.Mue_Lat_Max
  Gain{7..9,11} (4 alike) : Gain  Gain=-1
  Gain2 : Gain
  Gain3 : Gain
  Gain6 : Gain  Gain=d
  Judge Static Friction : Subsystem
  Product{,1,4..5,9..10} (6 alike) : Product
  Product2 : Product  Multiplication=Matrix(*)
  Selector : Selector  InputPortWidth=3  IndexOptions=Index vector (dialog)  Indices=[1]  OutputSizes=1
  Terminator : Terminator
  TrafoMX Backrotate Z : BaseLibrary/TrafoMX Backrotate Z
  Vector Concatenate : Concatenate  NumInputs=3  Mode=Multidimensional array
  FOR_GearLeg_R_0 : Outport  Unit=N  PortDimensions=[3,1]
  Static_Flag : Outport  Port=2  PortDimensions=[1]
  wires:
  Gain11/1 -> Product10/1
  Product10/1 -> Vector Concatenate/3, Product1/2, Judge Static Friction/4(Fdown), Product/2
  Product4/1 -> Gain7/1
  Gain9/1 -> Add2/2, Display10/1  "Fd"
  1-D Lookup Table/1 -> Product4/1
  Compare To Zero1/1 -> Product9/2, Product10/2
  Discrete-Time Integrator2/1 -> Gain8/1, Product4/2, Display6/1  "x1"
  Gain8/1 -> 1-D Lookup Table/1
  Gain7/1 -> Add2/1, Display9/1  "Fc"
  Gain6/1 -> Gain9/1
  Bus Selector/2 -> Compare To Zero1/1, Display4/1  "<POS_Alt_GearStrut>"
  Bus Selector/1 -> Product9/1, Display3/1  "<VEL_Alt_Dot_GearStrut>"
  Product9/1 -> Gain6/1, Discrete-Time Integrator2/1, Display5/1  "x1d"
  Judge Static Friction/2(Static_Flag) -> Static_Flag/1
  Judge Static Friction/1(FOR_GearLeg_R_0) -> FOR_GearLeg_R_0/1
  Gear_Kinematics/1 -> Bus Selector/1, Friction Model/1, Bus Selector1/1, Judge Static Friction/3(Gear_Kinematics)
  Kin_input/1 -> Judge Static Friction/1(Kin_input)
  FOR_WithoutGear_B/1 -> Judge Static Friction/2(FOR_WithoutGear_B)
  RB_States/1 -> Terminator/1
  " Sign "/1 -> Product5/2
  Product5/1 -> Vector Concatenate/1  "Flong"
  Product/1 -> Product5/1
  Add2/1 -> Gain11/1  "Fdown"
  Product1/1 -> Vector Concatenate/2  "Flat"
  Selector/1 -> " Sign "/1
  Product2/1 -> Judge Static Friction/5(FOR_GearLeg_R_0dyn)  "FOR_GearLeg_R_0dyn"
  Bus Selector/3 -> Selector/1  "<VEL_K_Gear_Local>"
  Gain2/1 -> Product1/1
  Gain3/1 -> Product/1
  Bus Selector1/1 -> TrafoMX Backrotate Z/1  "<Tire_Heading>"
  TrafoMX Backrotate Z/1 -> Product2/1
  Vector Concatenate/1 -> Product2/2
  Friction Model/2 -> Gain2/1
  Friction Model/1 -> Gain3/1

== system GearLibrary/Friction Model ==
  note: when velocity is small， forbidden lateral gear force
  Gear_Kinematics : Inport  OutDataTypeStr=Bus: GearKinematics_BUS
  Abs : Abs
  Bus Selector1 : BusSelector  OutputSignals=Rel_Angle_SpeedTire
  Bus Selector3 : BusSelector  OutputSignals=VEL_K_Gear_Local
  "Dead Zone " : DeadZone  LowerValue=0  SaturateOnIntegerOverflow=on
  Max. Lateral Friction : Saturate  UpperLimit=Mue_Lat_Max  LowerLimit=-Mue_Lat_Max
  Mue lateral per deflection : Constant  Value=Mue_Lat_per_Slip
  Product : Product
  Product1 : Product
  Rolling Friction : Constant  Value=Mue_Roll
  Saturation : Saturate  UpperLimit=1  LowerLimit=-1
  Selector1 : Selector  InputPortWidth=3  IndexOptions=Index vector (dialog)  Indices=[1]  OutputSizes=1
  Mue_Long : Outport
  Mue_Lat : Outport  Port=2
  wires:
  Gear_Kinematics/1 -> Bus Selector3/1, Bus Selector1/1
  Rolling Friction/1 -> Mue_Long/1
  Bus Selector1/1 -> Product/1  "<Rel_Angle_SpeedTire>"
  Product/1 -> Max. Lateral Friction/1
  Max. Lateral Friction/1 -> Mue_Lat/1  "Mue_lat"
  Selector1/1 -> Abs/1
  Abs/1 -> "Dead Zone "/1
  Saturation/1 -> Product1/2
  "Dead Zone "/1 -> Saturation/1
  Product1/1 -> Product/2
  Mue lateral per deflection/1 -> Product1/1
  Bus Selector3/1 -> Selector1/1  "<VEL_K_Gear_Local>"

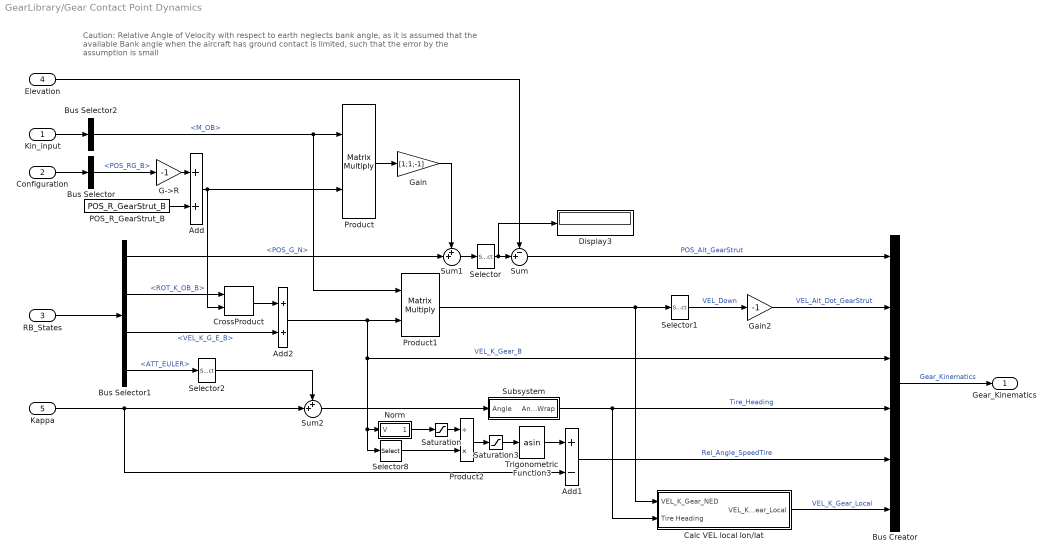
== system GearLibrary/Gear Contact Point Dynamics ==
  note: Caution: Relative Angle of Velocity with respect to earth neglects bank angle,
      | as it is assumed that the available Bank angle when the aircraft has ground contact is limited,
      | such that the error by the assumption is small
  Kin_input : Inport  OutDataTypeStr=Bus: Kin_input_BUS
  Configuration : Inport  Port=2  OutDataTypeStr=Bus: Configuration_BUS
  RB_States : Inport  Port=3  OutDataTypeStr=Bus: RB_State_BUS
  Elevation : Inport  Port=4  Unit=m  PortDimensions=[1,1]
  Kappa : Inport  Port=5  Unit=rad  PortDimensions=[1,1]
  Add : Sum  Inputs=2
  Add1 : Sum  Inputs=+-
  Add2 : Sum  Inputs=2
  Bus Creator : BusCreator  Inputs='POS_Alt_GearStrut','VEL_Alt_Dot_GearStrut','VEL_K_Gear_B','Tire_Heading','Rel_Angle_SpeedTire','VEL_K_Gear_Local'  OutDataTypeStr=Bus: GearKinematics_BUS  NonVirtualBus=on
  Bus Selector : BusSelector  OutputSignals=POS_RG_B
  Bus Selector1 : BusSelector  OutputSignals=POS_G_N,ROT_K_OB_B,VEL_K_G_E_B,ATT_EULER
  Bus Selector2 : BusSelector  OutputSignals=M_OB
  Calc VEL local lon/lat : Subsystem
  CrossProduct : BaseLibrary/CrossProduct
  Display3 : Display
  G->R : Gain  Gain=-1
  Gain : Gain  Gain=[1;1;-1]
  Gain2 : Gain  Gain=-1
  Norm : Subsystem
  POS_R_GearStrut_B : Constant  Value=POS_R_GearStrut_B  VectorParams1D=off
  Product : Product  Multiplication=Matrix(*)
  Product1 : Product  Multiplication=Matrix(*)
  Product2 : Product  Inputs=/*
  Saturation : Saturate  UpperLimit=inf  LowerLimit=0.5
  Saturation3 : Saturate  UpperLimit=1  LowerLimit=-1
  Selector : Selector  InputPortWidth=3  IndexOptions=Index vector (dialog)  Indices=[3]  OutputSizes=1
  Selector1 : Selector  InputPortWidth=3  IndexOptions=Index vector (dialog)  Indices=[3]  OutputSizes=1
  Selector2 : Selector  InputPortWidth=3  IndexOptions=Index vector (dialog)  Indices=[3]  OutputSizes=1
  Selector8 : Selector  InputPortWidth=3  IndexOptions=Index vector (dialog)  Indices=[2]  OutputSizes=1
  Subsystem : Subsystem
  Sum : Sum  Inputs=-+|
  Sum1 : Sum  Inputs=++|
  Sum2 : Sum  Inputs=++|
  Trigonometric Function3 : Trigonometry  Operator=asin
  Gear_Kinematics : Outport  OutDataTypeStr=Bus: GearKinematics_BUS
  wires:
  Gain2/1 -> Bus Creator/2  "VEL_Alt_Dot_GearStrut"
  Gain/1 -> Sum1/1
  Configuration/1 -> Bus Selector/1
  Bus Selector2/1 -> Product1/1, Product/1  "<M_OB>"
  Add/1 -> CrossProduct/2, Product/2
  POS_R_GearStrut_B/1 -> Add/2
  Product/1 -> Gain/1
  Sum1/1 -> Selector/1
  Bus Selector/1 -> G->R/1  "<POS_RG_B>"
  Bus Selector1/1 -> Sum1/2  "<POS_G_N>"
  Kin_input/1 -> Bus Selector2/1
  RB_States/1 -> Bus Selector1/1
  G->R/1 -> Add/1
  Bus Selector1/2 -> CrossProduct/1  "<ROT_K_OB_B>"
  Bus Selector1/3 -> Add2/2  "<VEL_K_G_E_B>"
  CrossProduct/1 -> Add2/1
  Add2/1 -> Product1/2, Norm/1(V), Selector8/1, Bus Creator/3  "VEL_K_Gear_B"
  Product1/1 -> Calc VEL local lon/lat/1(VEL_K_Gear_NED), Selector1/1
  Elevation/1 -> Sum/1
  Selector/1 -> Display3/1, Sum/2
  Sum/1 -> Bus Creator/1  "POS_Alt_GearStrut"
  Selector1/1 -> Gain2/1  "VEL_Down"
  Bus Creator/1 -> Gear_Kinematics/1  "Gear_Kinematics"
  Norm/1(||V||) -> Saturation/1
  Saturation/1 -> Product2/1
  Product2/1 -> Saturation3/1
  Saturation3/1 -> Trigonometric Function3/1
  Trigonometric Function3/1 -> Add1/1
  Bus Selector1/4 -> Selector2/1  "<ATT_EULER>"
  Selector2/1 -> Sum2/1
  Sum2/1 -> Subsystem/1(Angle)
  Add1/1 -> Bus Creator/5  "Rel_Angle_SpeedTire"
  Subsystem/1(AngleWrap) -> Calc VEL local lon/lat/2(Tire Heading), Bus Creator/4  "Tire_Heading"
  Selector8/1 -> Product2/2
  Kappa/1 -> Sum2/2, Add1/2
  Calc VEL local lon/lat/1(VEL_K_Gear_Local) -> Bus Creator/6  "VEL_K_Gear_Local"

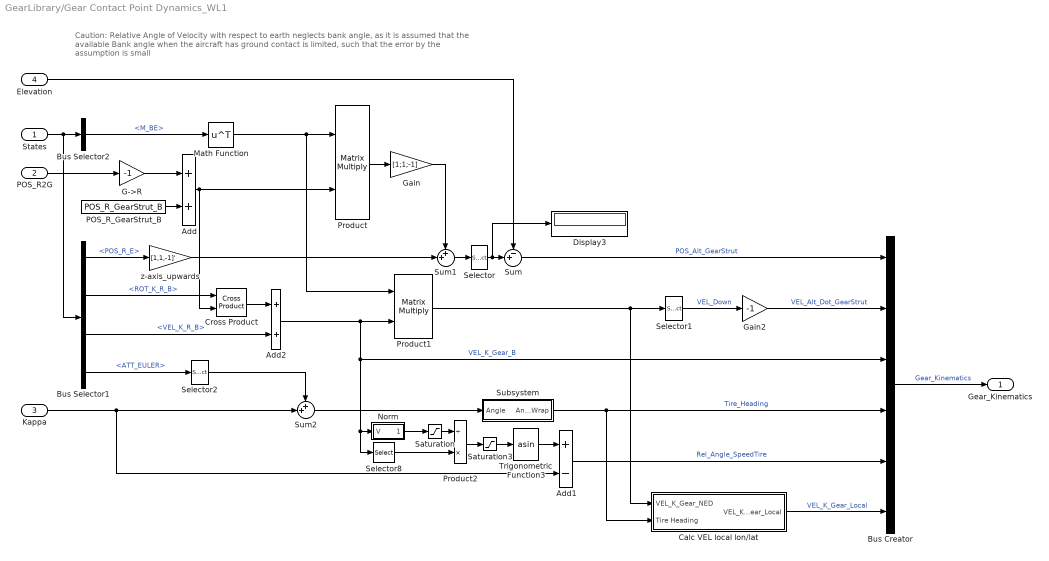
== system GearLibrary/Gear Contact Point Dynamics_WL1 ==
  note: Caution: Relative Angle of Velocity with respect to earth neglects bank angle,
      | as it is assumed that the available Bank angle when the aircraft has ground contact is limited,
      | such that the error by the assumption is small
  States : Inport  OutDataTypeStr=Bus: States_BUS
  POS_R2G : Inport  Port=2
  Kappa : Inport  Port=3  Unit=rad  PortDimensions=[1,1]
  Elevation : Inport  Port=4  Unit=m  PortDimensions=[1,1]
  Add : Sum  Inputs=2
  Add1 : Sum  Inputs=+-
  Add2 : Sum  Inputs=2
  Bus Creator : BusCreator  Inputs='POS_Alt_GearStrut','VEL_Alt_Dot_GearStrut','VEL_K_Gear_B','Tire_Heading','Rel_Angle_SpeedTire','VEL_K_Gear_Local'  OutDataTypeStr=Bus: GearKinematics_BUS  NonVirtualBus=on
  Bus Selector1 : BusSelector  OutputSignals=POS_R_E,ROT_K_R_B,VEL_K_R_B,ATT_EULER
  Bus Selector2 : BusSelector  OutputSignals=M_BE
  Calc VEL local lon/lat : Subsystem
  Cross Product : vrlib/Utilities/Cross Product
      settings: SourceProductBaseCode=VR
  Display3 : Display
  G->R : Gain  Gain=-1
  Gain : Gain  Gain=[1;1;-1]
  Gain2 : Gain  Gain=-1
  Math Function : Math  Operator=transpose  SaturateOnIntegerOverflow=on
  Norm : Subsystem
  POS_R_GearStrut_B : Constant  Value=POS_R_GearStrut_B  VectorParams1D=off
  Product : Product  Multiplication=Matrix(*)
  Product1 : Product  Multiplication=Matrix(*)
  Product2 : Product  Inputs=/*
  Saturation : Saturate  UpperLimit=inf  LowerLimit=0.5
  Saturation3 : Saturate  UpperLimit=1  LowerLimit=-1
  Selector : Selector  InputPortWidth=3  IndexOptions=Index vector (dialog)  Indices=[3]  OutputSizes=1
  Selector1 : Selector  InputPortWidth=3  IndexOptions=Index vector (dialog)  Indices=[3]  OutputSizes=1
  Selector2 : Selector  InputPortWidth=3  IndexOptions=Index vector (dialog)  Indices=[3]  OutputSizes=1
  Selector8 : Selector  InputPortWidth=3  IndexOptions=Index vector (dialog)  Indices=[2]  OutputSizes=1
  Subsystem : Subsystem
  Sum : Sum  Inputs=-+|
  Sum1 : Sum  Inputs=++|
  Sum2 : Sum  Inputs=++|
  Trigonometric Function3 : Trigonometry  Operator=asin
  z-axis_upwards : Gain  Gain=[1,1,-1]'
  Gear_Kinematics : Outport  OutDataTypeStr=Bus: GearKinematics_BUS
  wires:
  Calc VEL local lon/lat/1(VEL_K_Gear_Local) -> Bus Creator/6  "VEL_K_Gear_Local"
  Kappa/1 -> Add1/2, Sum2/2
  Selector8/1 -> Product2/2
  Subsystem/1(AngleWrap) -> Bus Creator/4, Calc VEL local lon/lat/2(Tire Heading)  "Tire_Heading"
  Add1/1 -> Bus Creator/5  "Rel_Angle_SpeedTire"
  Sum2/1 -> Subsystem/1(Angle)
  Selector2/1 -> Sum2/1
  Bus Selector1/4 -> Selector2/1  "<ATT_EULER>"
  Trigonometric Function3/1 -> Add1/1
  Saturation3/1 -> Trigonometric Function3/1
  Product2/1 -> Saturation3/1
  Saturation/1 -> Product2/1
  Norm/1(||V||) -> Saturation/1
  Bus Creator/1 -> Gear_Kinematics/1  "Gear_Kinematics"
  Selector1/1 -> Gain2/1  "VEL_Down"
  Sum/1 -> Bus Creator/1  "POS_Alt_GearStrut"
  Selector/1 -> Sum/2, Display3/1
  Elevation/1 -> Sum/1
  Product1/1 -> Selector1/1, Calc VEL local lon/lat/1(VEL_K_Gear_NED)
  Add2/1 -> Bus Creator/3, Selector8/1, Norm/1(V), Product1/2  "VEL_K_Gear_B"
  Cross Product/1 -> Add2/1
  Bus Selector1/3 -> Add2/2  "<VEL_K_R_B>"
  Bus Selector1/2 -> Cross Product/1  "<ROT_K_R_B>"
  G->R/1 -> Add/1
  States/1 -> Bus Selector1/1, Bus Selector2/1
  Bus Selector1/1 -> z-axis_upwards/1  "<POS_R_E>"
  POS_R2G/1 -> G->R/1
  Sum1/1 -> Selector/1
  Product/1 -> Gain/1
  POS_R_GearStrut_B/1 -> Add/2
  Add/1 -> Cross Product/2, Product/2
  Bus Selector2/1 -> Math Function/1  "<M_BE>"
  Gain/1 -> Sum1/1
  Gain2/1 -> Bus Creator/2  "VEL_Alt_Dot_GearStrut"
  Math Function/1 -> Product/1, Product1/1
  z-axis_upwards/1 -> Sum1/2

== system GearLibrary/Gear Strut ==
  Kin_input : Inport  OutDataTypeStr=Bus: Kin_input_BUS
  Configuration : Inport  Port=2  OutDataTypeStr=Bus: Configuration_BUS
  RB_States : Inport  Port=3  OutDataTypeStr=Bus: RB_State_BUS
  Elevation : Inport  Port=4  Unit=m  PortDimensions=1
  Kappa : Inport  Port=5  Unit=rad  PortDimensions=1
  FOR_WithouGear_B : Inport  Port=6
  Bus Selector : BusSelector  OutputSignals=Rel_Angle_SpeedTire
  Forces and Moments Body : GearLibrary/Forces and Moments Body  POS_R_GearStrut_B=Strut.POS_R_GearStrut_B
  Forces in Contact Point : GearLibrary/Forces in Contact Point  h_StrutUndeflected=Strut.h_StrutUndeflected  c=Strut.c  d=Strut.d  ct=Strut.ct  dt=Strut.dt  FOR_MaxDamp=Strut.FOR_MaxDamp  FOR_MaxSpring=Strut.FOR_MaxSpring  Mue_Roll=Strut.Mue_Roll  Mue_Lat_per_Slip=Strut.Mue_Lat_per_Slip  Mue_Lat_Max=Strut.Mue_Lat_Max  Compress_LengthMax=Strut.Compress_LengthMax  Mue_Static=Strut.Mue_Static
  Gear Contact Point Dynamics : GearLibrary/Gear Contact Point Dynamics  POS_R_GearStrut_B=Strut.POS_R_GearStrut_B
  FOR_GearLeg_R_B : Outport  Unit=N  PortDimensions=[3,1]
  MOM_GearLeg_R_B : Outport  Port=2  Unit=N*m  PortDimensions=[3,1]
  Rel_Angle_SpeedTire : Outport  Port=3  Unit=rad  PortDimensions=[1]
  Static Flag : Outport  Port=4  PortDimensions=[1]
  wires:
  Forces in Contact Point/1 -> Forces and Moments Body/2
  Configuration/1 -> Gear Contact Point Dynamics/2
  Elevation/1 -> Gear Contact Point Dynamics/4
  Kappa/1 -> Gear Contact Point Dynamics/5
  Forces and Moments Body/1 -> FOR_GearLeg_R_B/1  "FOR_GearLeg_R_B"
  Forces and Moments Body/2 -> MOM_GearLeg_R_B/1  "MOM_GearLeg_R_B"
  RB_States/1 -> Forces in Contact Point/3, Gear Contact Point Dynamics/3
  Kin_input/1 -> Gear Contact Point Dynamics/1, Forces and Moments Body/1, Forces in Contact Point/1
  FOR_WithouGear_B/1 -> Forces in Contact Point/4
  Gear Contact Point Dynamics/1 -> Bus Selector/1, Forces in Contact Point/2
  Bus Selector/1 -> Rel_Angle_SpeedTire/1  "<Rel_Angle_SpeedTire>"
  Forces in Contact Point/2 -> Static Flag/1

== system GearLibrary/Gear Strut_WL1 ==
  States : Inport  OutDataTypeStr=Bus: States_BUS
  POS_R2G : Inport  Port=2
  Kappa : Inport  Port=3  Unit=rad  PortDimensions=1
  Elevation : Inport  Port=4  Unit=m  PortDimensions=1
  FOR_WithouGear_B : Inport  Port=5
  Bus Selector : BusSelector  OutputSignals=Rel_Angle_SpeedTire
  Forces and Moments Body_WL1 : GearLibrary/Forces and Moments Body_WL1  POS_R_GearStrut_B=Strut.POS_R_GearStrut_B
  Forces in Contact Point_WL1 : GearLibrary/Forces in Contact Point_WL1  h_StrutUndeflected=Strut.h_StrutUndeflected  c=Strut.c  d=Strut.d  ct=Strut.ct  dt=Strut.dt  FOR_MaxDamp=Strut.FOR_MaxDamp  FOR_MaxSpring=Strut.FOR_MaxSpring  Mue_Roll=Strut.Mue_Roll  Mue_Lat_per_Slip=Strut.Mue_Lat_per_Slip  Mue_Lat_Max=Strut.Mue_Lat_Max  Compress_LengthMax=Strut.Compress_LengthMax  Mue_Static=Strut.Mue_Static  Compress_LengthMax_Tire=Strut.Compress_LengthMax_Tire
  Gear Contact Point Dynamics_WL1 : GearLibrary/Gear Contact Point Dynamics_WL1  POS_R_GearStrut_B=Strut.POS_R_GearStrut_B
  FOR_GearLeg_R_B : Outport  Unit=N  PortDimensions=[3,1]
  MOM_GearLeg_R_B : Outport  Port=2  Unit=N*m  PortDimensions=[3,1]
  Rel_Angle_SpeedTire : Outport  Port=3  Unit=rad  PortDimensions=[1]
  Static Flag : Outport  Port=4  PortDimensions=[1]
  wires:
  Forces in Contact Point_WL1/1 -> Forces and Moments Body_WL1/2
  Forces and Moments Body_WL1/1 -> FOR_GearLeg_R_B/1  "FOR_GearLeg_R_B"
  Forces and Moments Body_WL1/2 -> MOM_GearLeg_R_B/1  "MOM_GearLeg_R_B"
  States/1 -> Gear Contact Point Dynamics_WL1/1, Forces in Contact Point_WL1/1, Forces and Moments Body_WL1/1
  FOR_WithouGear_B/1 -> Forces in Contact Point_WL1/3
  Gear Contact Point Dynamics_WL1/1 -> Bus Selector/1, Forces in Contact Point_WL1/2
  Bus Selector/1 -> Rel_Angle_SpeedTire/1  "<Rel_Angle_SpeedTire>"
  Forces in Contact Point_WL1/2 -> Static Flag/1
  POS_R2G/1 -> Gear Contact Point Dynamics_WL1/2
  Kappa/1 -> Gear Contact Point Dynamics_WL1/3
  Elevation/1 -> Gear Contact Point Dynamics_WL1/4

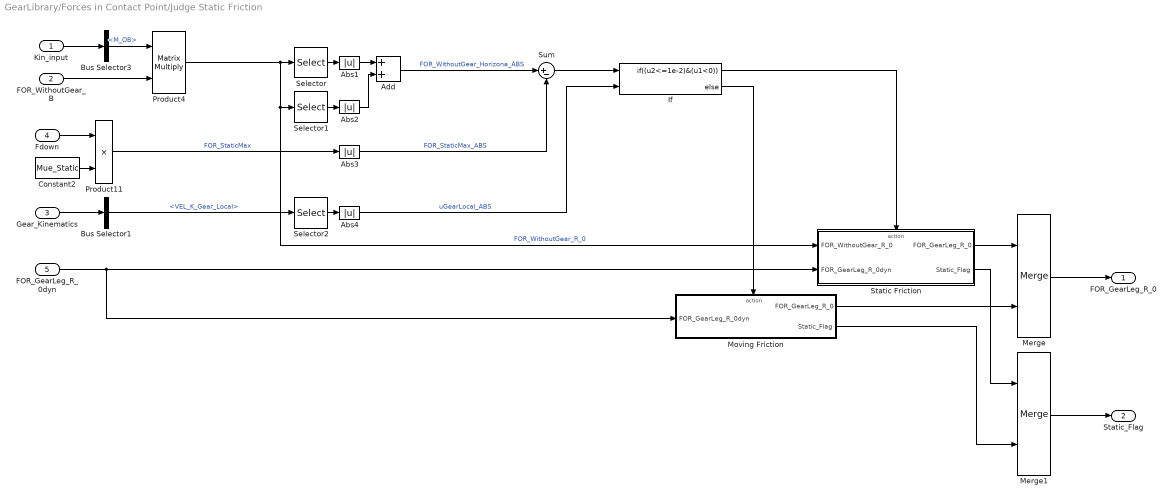
== system GearLibrary/Forces in Contact Point/Judge Static Friction ==
  Kin_input : Inport  OutDataTypeStr=Bus: Kin_input_BUS
  FOR_WithoutGear_B : Inport  Port=2  Unit=N  PortDimensions=[3 1]
  Gear_Kinematics : Inport  Port=3  OutDataTypeStr=Bus: GearKinematics_BUS
  Fdown : Inport  Port=4
  FOR_GearLeg_R_0dyn : Inport  Port=5
  Abs{1..4} (4 alike) : Abs
  Add : Sum
  Bus Selector1 : BusSelector  OutputSignals=VEL_K_Gear_Local
  Bus Selector3 : BusSelector  OutputSignals=M_OB
  Constant2 : Constant  Value=Mue_Static
  If : If  NumInputs=2  IfExpression=(u2<=1e-2)&(u1<0)
  Merge : Merge
  Merge1 : Merge
  Moving Friction : Subsystem  TreatAsAtomicUnit=on
  Product11 : Product
  Product4 : Product  Multiplication=Matrix(*)
  Selector : Selector  InputPortWidth=3  IndexOptions=Index vector (dialog)  Indices=[1]  OutputSizes=1
  Selector1 : Selector  InputPortWidth=3  IndexOptions=Index vector (dialog)  Indices=[2]  OutputSizes=1
  Selector2 : Selector  InputPortWidth=3  IndexOptions=Index vector (dialog)  Indices=[1]  OutputSizes=1
  "Static Friction " : Subsystem  TreatAsAtomicUnit=on
  Sum : Sum  Inputs=|+-
  FOR_GearLeg_R_0 : Outport  Unit=N  PortDimensions=[3,1]
  Static_Flag : Outport  Port=2  PortDimensions=[1]
  wires:
  Fdown/1 -> Product11/1
  Constant2/1 -> Product11/2
  Product11/1 -> Abs3/1  "FOR_StaticMax"
  Kin_input/1 -> Bus Selector3/1
  Bus Selector3/1 -> Product4/1  "<M_OB>"
  FOR_WithoutGear_B/1 -> Product4/2
  Product4/1 -> "Static Friction "/1(FOR_WithoutGear_R_0), Selector1/1, Selector/1  "FOR_WithoutGear_R_0"
  Add/1 -> Sum/1  "FOR_WithoutGear_Horizona_ABS"
  Abs1/1 -> Add/1
  Selector/1 -> Abs1/1
  Selector1/1 -> Abs2/1
  Abs2/1 -> Add/2
  Abs3/1 -> Sum/2  "FOR_StaticMax_ABS"
  Sum/1 -> If/1
  Gear_Kinematics/1 -> Bus Selector1/1
  Bus Selector1/1 -> Selector2/1  "<VEL_K_Gear_Local>"
  Selector2/1 -> Abs4/1
  Abs4/1 -> If/2  "uGearLocal_ABS"
  If/1 -> "Static Friction "/Action
  "Static Friction "/1(FOR_GearLeg_R_0) -> Merge/1
  If/2 -> Moving Friction/Action
  FOR_GearLeg_R_0dyn/1 -> "Static Friction "/2(FOR_GearLeg_R_0dyn), Moving Friction/1(FOR_GearLeg_R_0dyn)
  Moving Friction/1(FOR_GearLeg_R_0) -> Merge/2
  Merge/1 -> FOR_GearLeg_R_0/1
  Moving Friction/2(Static_Flag) -> Merge1/2
  Merge1/1 -> Static_Flag/1
  "Static Friction "/2(Static_Flag) -> Merge1/1

== system GearLibrary/Forces in Contact Point_WL1/If Action Subsystem ==
  Action Port : ActionPort
  Constant : Constant  Value=0
  Fz=0 : Outport
  wires:
  Constant/1 -> Fz=0/1

== system GearLibrary/Forces in Contact Point_WL1/If Action Subsystem1 ==
  v : Inport
  x : Inport  Port=2
  Action Port : ActionPort  InitializeStates=reset
  " " : Saturate  UpperLimit=FOR_MaxDamp  LowerLimit=-FOR_MaxDamp
  Add : Sum
  Gain7 : Gain  Gain=d
  Gain8 : Gain  Gain=c
  Saturation : Saturate  UpperLimit=Compress_LengthMax*c  LowerLimit=-Compress_LengthMax*c
  Fz : Outport
  wires:
  " "/1 -> Add/1  "Fd"
  Gain7/1 -> " "/1
  Saturation/1 -> Add/2  "Fc"
  Add/1 -> Fz/1  "Fz1"
  Gain8/1 -> Saturation/1
  x/1 -> Gain8/1  "x1"
  v/1 -> Gain7/1  "x1dot"

== system GearLibrary/Forces in Contact Point_WL1/If Action Subsystem2 ==
  v : Inport
  x : Inport  Port=2
  Action Port : ActionPort  InitializeStates=reset
  Add : Sum
  Constant : Constant  Value=Compress_LengthMax
  Constant1 : Constant  Value=Compress_LengthMax*c
  Fc2tox2 : Lookup_n-D  NumberOfTableDimensions=1  BreakpointsForDimension1=(linspace(0,Compress_LengthMax_Tire,30) * (9 * ct / Compress_LengthMax_Tire) + ct).*linspace(0,Compress_LengthMax_Tire,30)  Table=linspace(0,Compress_LengthMax_Tire,30)  InternalRulePriority=Speed  RndMeth=Simplest  InputSameDT=on
  Gain : Gain  Gain=-1
  Gain1 : Gain  Gain=-1
  Gain12 : Gain  Gain=dt
  Saturation : Saturate  UpperLimit=0  LowerLimit=-10*ct*Compress_LengthMax_Tire
  Sum : Sum  Inputs=|++
  Sum1 : Sum  Inputs=|+-
  x2toFc2 : Lookup_n-D  NumberOfTableDimensions=1  BreakpointsForDimension1=linspace(0,Compress_LengthMax_Tire,30)  Table=(linspace(0,Compress_LengthMax_Tire,30) * (9 * ct / Compress_LengthMax_Tire) + ct).*linspace(0,Compress_LengthMax_Tire,30)  InternalRulePriority=Speed  RndMeth=Simplest  InputSameDT=on
  Fz : Outport
  wires:
  Fc2tox2/1 -> Sum1/2
  Gain1/1 -> Saturation/1
  Gain/1 -> x2toFc2/1
  Sum1/1 -> Gain/1
  Constant1/1 -> Fc2tox2/1
  Add/1 -> Fz/1  "Fz2"
  Saturation/1 -> Add/2  "Fct"
  Gain12/1 -> Add/1  "Fdt"
  x2toFc2/1 -> Gain1/1
  Constant/1 -> Sum/2
  Sum/1 -> Sum1/1
  v/1 -> Gain12/1
  x/1 -> Sum/1

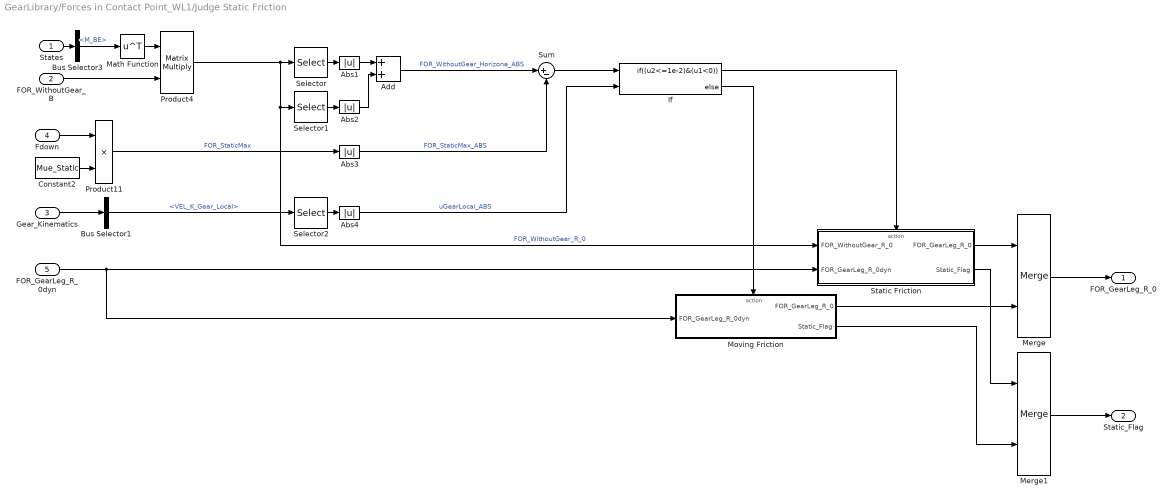
== system GearLibrary/Forces in Contact Point_WL1/Judge Static Friction ==
  States : Inport  OutDataTypeStr=Bus: States_BUS
  FOR_WithoutGear_B : Inport  Port=2  Unit=N  PortDimensions=[3 1]
  Gear_Kinematics : Inport  Port=3  OutDataTypeStr=Bus: GearKinematics_BUS
  Fdown : Inport  Port=4
  FOR_GearLeg_R_0dyn : Inport  Port=5
  Abs{1..4} (4 alike) : Abs
  Add : Sum
  Bus Selector1 : BusSelector  OutputSignals=VEL_K_Gear_Local
  Bus Selector3 : BusSelector  OutputSignals=M_BE
  Constant2 : Constant  Value=Mue_Static
  If : If  NumInputs=2  IfExpression=(u2<=1e-2)&(u1<0)
  Math Function : Math  Operator=transpose  SaturateOnIntegerOverflow=on
  Merge : Merge
  Merge1 : Merge
  Moving Friction : Subsystem  TreatAsAtomicUnit=on
  Product11 : Product
  Product4 : Product  Multiplication=Matrix(*)
  Selector : Selector  InputPortWidth=3  IndexOptions=Index vector (dialog)  Indices=[1]  OutputSizes=1
  Selector1 : Selector  InputPortWidth=3  IndexOptions=Index vector (dialog)  Indices=[2]  OutputSizes=1
  Selector2 : Selector  InputPortWidth=3  IndexOptions=Index vector (dialog)  Indices=[1]  OutputSizes=1
  "Static Friction " : Subsystem  TreatAsAtomicUnit=on
  Sum : Sum  Inputs=|+-
  FOR_GearLeg_R_0 : Outport  Unit=N  PortDimensions=[3,1]
  Static_Flag : Outport  Port=2  PortDimensions=[1]
  wires:
  Fdown/1 -> Product11/1
  Constant2/1 -> Product11/2
  Product11/1 -> Abs3/1  "FOR_StaticMax"
  States/1 -> Bus Selector3/1
  Bus Selector3/1 -> Math Function/1  "<M_BE>"
  FOR_WithoutGear_B/1 -> Product4/2
  Product4/1 -> "Static Friction "/1(FOR_WithoutGear_R_0), Selector1/1, Selector/1  "FOR_WithoutGear_R_0"
  Add/1 -> Sum/1  "FOR_WithoutGear_Horizona_ABS"
  Abs1/1 -> Add/1
  Selector/1 -> Abs1/1
  Selector1/1 -> Abs2/1
  Abs2/1 -> Add/2
  Abs3/1 -> Sum/2  "FOR_StaticMax_ABS"
  Sum/1 -> If/1
  Gear_Kinematics/1 -> Bus Selector1/1
  Bus Selector1/1 -> Selector2/1  "<VEL_K_Gear_Local>"
  Selector2/1 -> Abs4/1
  Abs4/1 -> If/2  "uGearLocal_ABS"
  If/1 -> "Static Friction "/Action
  "Static Friction "/1(FOR_GearLeg_R_0) -> Merge/1
  If/2 -> Moving Friction/Action
  FOR_GearLeg_R_0dyn/1 -> "Static Friction "/2(FOR_GearLeg_R_0dyn), Moving Friction/1(FOR_GearLeg_R_0dyn)
  Moving Friction/1(FOR_GearLeg_R_0) -> Merge/2
  Merge/1 -> FOR_GearLeg_R_0/1
  Moving Friction/2(Static_Flag) -> Merge1/2
  Merge1/1 -> Static_Flag/1
  "Static Friction "/2(Static_Flag) -> Merge1/1
  Math Function/1 -> Product4/1

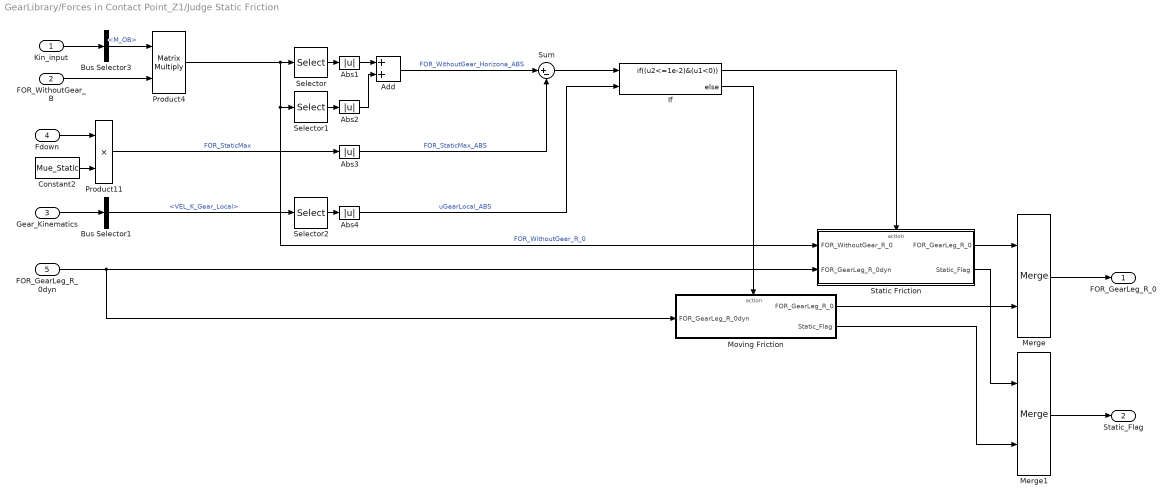
== system GearLibrary/Forces in Contact Point_Z1/Judge Static Friction ==
  Kin_input : Inport  OutDataTypeStr=Bus: Kin_input_BUS
  FOR_WithoutGear_B : Inport  Port=2  Unit=N  PortDimensions=[3 1]
  Gear_Kinematics : Inport  Port=3  OutDataTypeStr=Bus: GearKinematics_BUS
  Fdown : Inport  Port=4
  FOR_GearLeg_R_0dyn : Inport  Port=5
  Abs{1..4} (4 alike) : Abs
  Add : Sum
  Bus Selector1 : BusSelector  OutputSignals=VEL_K_Gear_Local
  Bus Selector3 : BusSelector  OutputSignals=M_OB
  Constant2 : Constant  Value=Mue_Static  SampleTime=Tss
  If : If  NumInputs=2  IfExpression=(u2<=1e-2)&(u1<0)
  Merge : Merge
  Merge1 : Merge
  Moving Friction : Subsystem  TreatAsAtomicUnit=on
  Product11 : Product
  Product4 : Product  Multiplication=Matrix(*)
  Selector : Selector  InputPortWidth=3  IndexOptions=Index vector (dialog)  Indices=[1]  OutputSizes=1
  Selector1 : Selector  InputPortWidth=3  IndexOptions=Index vector (dialog)  Indices=[2]  OutputSizes=1
  Selector2 : Selector  InputPortWidth=3  IndexOptions=Index vector (dialog)  Indices=[1]  OutputSizes=1
  "Static Friction " : Subsystem  TreatAsAtomicUnit=on
  Sum : Sum  Inputs=|+-
  FOR_GearLeg_R_0 : Outport  Unit=N  PortDimensions=[3,1]
  Static_Flag : Outport  Port=2  PortDimensions=[1]
  wires:
  Fdown/1 -> Product11/1
  Constant2/1 -> Product11/2
  Product11/1 -> Abs3/1  "FOR_StaticMax"
  Kin_input/1 -> Bus Selector3/1
  Bus Selector3/1 -> Product4/1  "<M_OB>"
  FOR_WithoutGear_B/1 -> Product4/2
  Product4/1 -> "Static Friction "/1(FOR_WithoutGear_R_0), Selector1/1, Selector/1  "FOR_WithoutGear_R_0"
  Add/1 -> Sum/1  "FOR_WithoutGear_Horizona_ABS"
  Abs1/1 -> Add/1
  Selector/1 -> Abs1/1
  Selector1/1 -> Abs2/1
  Abs2/1 -> Add/2
  Abs3/1 -> Sum/2  "FOR_StaticMax_ABS"
  Sum/1 -> If/1
  Gear_Kinematics/1 -> Bus Selector1/1
  Bus Selector1/1 -> Selector2/1  "<VEL_K_Gear_Local>"
  Selector2/1 -> Abs4/1
  Abs4/1 -> If/2  "uGearLocal_ABS"
  If/1 -> "Static Friction "/Action
  "Static Friction "/1(FOR_GearLeg_R_0) -> Merge/1
  If/2 -> Moving Friction/Action
  FOR_GearLeg_R_0dyn/1 -> "Static Friction "/2(FOR_GearLeg_R_0dyn), Moving Friction/1(FOR_GearLeg_R_0dyn)
  Moving Friction/1(FOR_GearLeg_R_0) -> Merge/2
  Merge/1 -> FOR_GearLeg_R_0/1
  Moving Friction/2(Static_Flag) -> Merge1/2
  Merge1/1 -> Static_Flag/1
  "Static Friction "/2(Static_Flag) -> Merge1/1

== system GearLibrary/Forces in Contact Point_Z2/If Action Subsystem ==
  Action Port : ActionPort  ActionType=then
  Constant : Constant  Value=0
  Fz=0 : Outport
  wires:
  Constant/1 -> Fz=0/1
